simulink model "SF040A_MotVel"  (R2013b)
settings: Solver=FixedStepDiscrete  SolverMode=SingleTasking  StartTime=0.0  StopTime=1  FixedStep=6.25E-5  RelTol=1e-3
values from neighbouring files (symbols this model uses):
  ARCHGLBPRM_2MILLISEC_SEC_F32 = DataDict.Constant    [SF040A_MotVel_DataDict.m]
  ARCHGLBPRM_2PI_ULS_F32 = DataDict.Constant    [SF040A_MotVel_DataDict.m]
  ARCHGLBPRM_FLOATZEROTHD_ULS_F32 = DataDict.Constant    [SF040A_MotVel_DataDict.m]
  ARCHGLBPRM_PI_ULS_F32 = DataDict.Constant    [SF040A_MotVel_DataDict.m]
  BITMASK16BIT_CNT_U32 = DataDict.Constant    [SF040A_MotVel_DataDict.m]
  BUFSIZE_CNT_U08 = DataDict.Constant    [SF040A_MotVel_DataDict.m]
  BUFSIZECOMBD_CNT_U08 = DataDict.Constant    [SF040A_MotVel_DataDict.m]
  MOTVELMAXININVAL_CNT_U08 = DataDict.Constant    [SF040A_MotVel_DataDict.m]
  SECTOMICROSEC_ULS_F32 = DataDict.Constant    [SF040A_MotVel_DataDict.m]
  SysGlbPrmSysKineRat = DataDict.ImprtdCal    [SF040A_MotVel_DataDict.m]
libraries: simulink x7, NxtrLim x3, FixdToFloat x1
(part 1 of 2)
settings Model: Creator=BZHF94  LastModifiedBy=bzhf94
settings SolverCC: AutoInsertRateTranBlk=on  InsertRTBMode=Always
settings DataIOCC: LimitDataPoints=off  SaveFormat=Structure  ReturnWorkspaceOutputs=on
settings OptimizationCC: BlockReduction=off  InlineParams=on  ZeroExternalMemoryAtStartup=off  ZeroInternalMemoryAtStartup=off  OptimizeModelRefInitCode=on  LifeSpan=1
settings DebuggingCC: SignalInfNanChecking=error  SignalRangeChecking=warning  UnderspecifiedInitializationDetection=Simplified  SolverPrmCheckMsg=error  InheritedTsInSrcMsg=error  DiscreteInheritContinuousMsg=error  SingleTaskRateTransMsg=error  TasksWithSamePriorityMsg=error  SigSpecEnsureSampleTimeMsg=error  CheckMatrixSingularityMsg=error  ParameterUnderflowMsg=error  ParameterPrecisionLossMsg=error  ParameterTunabilityLossMsg=error  FixptConstUnderflowMsg=warning  FixptConstOverflowMsg=warning  VectorMatrixConversionMsg=error  SignalLabelMismatchMsg=error  UnconnectedInputMsg=error  UnconnectedOutputMsg=error  UnconnectedLineMsg=error  SFcnCompatibilityMsg=error  UniqueDataStoreMsg=warning  BusObjectLabelMismatch=error  RootOutportRequireBusObject=error  AssertControl=DisableAll  ModelReferenceIOMsg=error  ModelReferenceVersionMismatchMessage=warning  ModelReferenceIOMismatchMessage=error  ModelReferenceCSMismatchMessage=warning  ModelReferenceDataLoggingMessage=error  StateNameClashWarn=warning  StrictBusMsg=ErrorOnBusTreatedAsVector  NonBusSignalsTreatedAsBus=error  SFUnexpectedBacktrackingDiag=error  SFInvalidInputDataAccessInChartInitDiag=error  SFNoUnconditionalDefaultTransitionDiag=error  SFTransitionOutsideNaturalParentDiag=error  SFUnconditionalTransitionShadowingDiag=error  SFUndirectedBroadcastEventsDiag=error
settings ModelReferenceCC: ModelReferenceNumInstancesAllowed=Single
settings RTWCC: SystemTargetFile=autosar.tlc  GenCodeOnly=on  TemplateMakefile=ert_default_tmf  Description=AUTOSAR  GenerateReport=on  ProcessScript=autosar_make_rtw_hook  LaunchReport=on
settings CodeAppCC: GenerateComments=off  IgnoreCustomStorageClasses=off  CustomSymbolStrType=$N$R$M  CustomSymbolStrBlkIO=$N$M  SimulinkBlockComments=off
settings STFCustomTargetCC: ParMdlRefBuildCompliant=on  CompOptLevelCompliant=on  IncludeMdlTerminateFcn=off  CombineOutputUpdateFcns=on  SuppressErrorStatus=on  ERTFirstTimeCompliant=on  ERTCustomFileBanners=on  SupportNonFinite=off  SupportComplex=off  SupportContinuousTime=off  SupportNonInlinedSFcns=off  MATLABClassNameForMDSCustomization=Simulink.SoftwareTarget.ERTCustomization  AutosarCompliant=on  GRTInterface=off  SystemTargetFile=autosar.tlc
settings ERTTargetCC: CodeReplacementLibrary=ANSI_C  ConcurrentExecutionCompliant=off  IncludeMdlTerminateFcn=off  SuppressErrorStatus=on  SupportNonFinite=off  SupportComplex=off  ModelStepFunctionPrototypeControlCompliant=off  CPPClassGenCompliant=off  AutosarCompliant=on  InlinedParameterPlacement=NonHierarchical  ERTCustomFileTemplate=example_file_process.tlc  EnableUserReplacementTypes=on

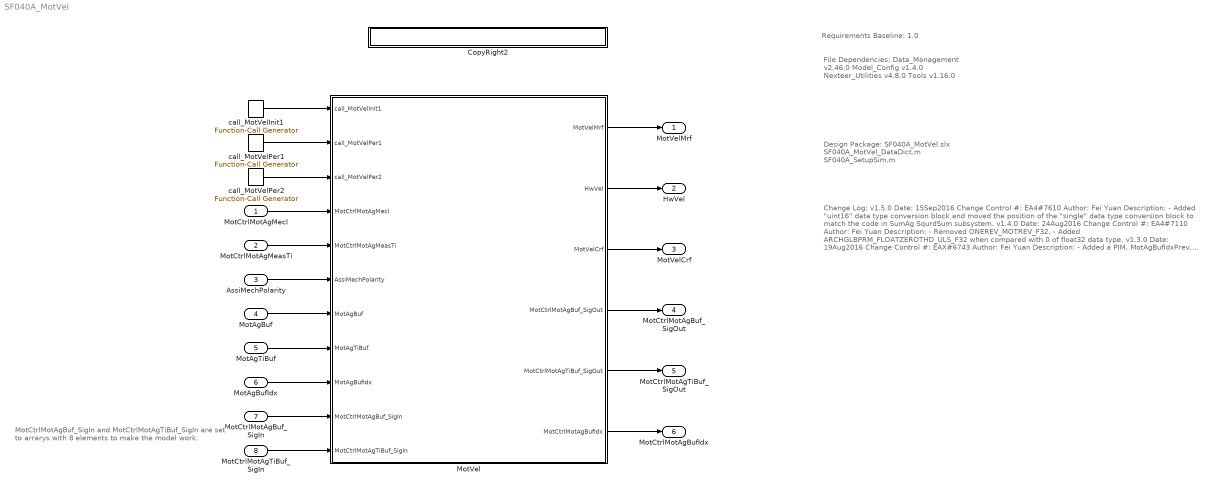
== system SF040A_MotVel ==
  note: MotCtrlMotAgBuf_SigIn and MotCtrlMotAgTiBuf_SigIn are
      | set to arrarys with 8 elements to make the model work.
  note: Change Log:
      |
      |
      | v1.5.0
      | Date: 15Sep2016
      | Change Control #: EA4#7610
      | Author: Fei Yuan
      | Description:
      | - Added "uint16" data type conversion block and moved the position of the
      |   "single" data type conversion block to match the code in SumAg SqurdSum
      |   subsystem.
      |
      | v1.4.0
      | Date: 24Aug2016
      | Change Control #: EA4#7110
      | Author: Fei Yuan
      | Description:
      | - Removed ONEREV_MOTREV_F32.
      | - Added ARCHGLBPRM_FLOATZEROTHD_ULS_F32 when compared with
      |   0 of float32 data type.
      |
      | v1.3.0
      | Date: 19Aug2016
      | Change Control #: EAX#6743
      | Author: Fei Yuan
      | Description:
      | - Added a PIM, MotAgBufIdxPrev, 3 constants, ARCHGLBPRM_PI_ULS_F32,
      |   BITCON_CNT_U32, BUFSIZE2_CNT_U08.
      | - Changed the index used for calculation MotAgRef and TiStampRef.
      | - Converted the time stamp data type from u32 to u16 before any calculation.
      | - Changed the location of conversion of MotAg from MotRev to MotRad, and
      |   MotAgTi from MicroSec to Sec.
      | - Removed constant ADJTISTAMPFAC_CNT_U08, HALFREV_MOTREV_F32.
      | - Changed constant MICROSECTOSEC_ULS_F32 to
      |    MICROSECTOSEC_ULS_F32.
      |
      |
      | v 1.2.0
      | Date: 08Jun2016
      | CR#: EA4#5936
      | Author: Fei Yuan
      | Description:
      | - Added data type conversion blocks to match the code.
      | - Changed the EngDT to u0p16 for dMotVelMotAgRef.
      | - Changed the EngDT to u0p16 and EngMax to 0.9999847412 for
      |   MotAgBufPrev.
      | - Changed the EngDT to u32 for MotAgTiBufPrev.
      | - MotCtrlMotAgBuf_SigIn and MotCtrlMotAgTiBuf_SigIn are set to
      |   arrarys with 8 elements to make the model work.
      |
      | v 1.1.0
      | Date: 13Apr2016
      | Change Control #: EA4#5282
      | Author: Fei Yuan
      | Description:
      | - Replaced MotCtrlMotAgBufPrev and MotCtrlMotAgTiBufPrev with 2 input
      |   signals, MotCtrlMotAgBuf and MotCtrlMotAgTiBuf.
      | - Moved 3 PIMs, SumTiStampBufStPrev, SumAgTiMotRevSecPrev and
      |   SqdSumTiStampPrev from the structure layer to the layer where they
      |   were used and deleted the definition in the data dictionary.
      | - Changed the PIMs names, IdxCntrPrev to MotAgBufIdx, and VelInitCntr
      |   to MotVelIninCntr.
      |
      | v 1.0.0
      | Date: 30Mar2016
      | Change Control #:  EA4#4986
      | Author: Fei Yuan
      | Description:
      |
      | - Initial release (copy over from SF040B v 1.1.0)
      | - Change the MotVelPer1.Context to 'Non-Rte' and MotVelPer1.TimeStep
      |   to 'MotorControl'.
      | - Change the EngInit of MotAgBuf, MotAgTiBuf
  note: File Dependencies:
      |
      | Data_Management v2.46.0
      | Model_Config v1.4.0
      | Nexteer_Utilities v4.8.0
      | Tools v1.16.0
  note: Requirements Baseline: 1.0
  note: Design Package:
      | SF040A_MotVel.slx
      | SF040A_MotVel_DataDict.m
      | SF040A_SetupSim.m
  MotCtrlMotAgMecl : Inport
  MotCtrlMotAgMeasTi : Inport  Port=2
  AssiMechPolarity : Inport  Port=3
  MotAgBuf : Inport  Port=4
  MotAgTiBuf : Inport  Port=5
  MotAgBufIdx : Inport  Port=6
  MotCtrlMotAgBuf_SigIn : Inport  Port=7  PortDimensions=8
  MotCtrlMotAgTiBuf_SigIn : Inport  Port=8  PortDimensions=8
  CopyRight2 : Subsystem  Description=|  mask(Copyright Information){none=on}
      | Copyright info block.                                               
      |                                                                     
      | Place copyright information at the top of every subsystem in design.
      mask prompts: none "No parameters"
      mask help: Place copyright information at the top of every subsystem in design.
      mask Display:
      | NxtrConf = 'Nexteer Confidential';
      | 
      | sys = bdroot; %handle for the current model ("system")
      | first = get_param(sys,'Created');
      | first = first(end-3:end);  %year is last four digits
      | 
      | last = get_param(sys,'LastModifiedDate');
      | if isempty(last)
      |     last = datestr(now,'yyyy');
      | else
      |     last = last(end-3:end);
      | end
      | 
      | if strcmp(first,last)
      |     fprintf('%s -- Copyright %s Nexteer',NxtrConf,first)
      | else
      |     fprintf('%s -- %s%s- %s Nexteer',NxtrConf,char(169),first,last)
      | end
  MotVel : Subsystem
  call_MotVelInit1 : simulink/Ports & Subsystems/Function-Call Generator  sample_time=0.002  numberOfIterations=1
  call_MotVelPer1 : simulink/Ports & Subsystems/Function-Call Generator  sample_time=0.0000625  numberOfIterations=1
  call_MotVelPer2 : simulink/Ports & Subsystems/Function-Call Generator  sample_time=.002  numberOfIterations=1
  MotVelMrf : Outport
  HwVel : Outport  Port=2
  MotVelCrf : Outport  Port=3
  MotCtrlMotAgBuf_SigOut : Outport  Port=4
  MotCtrlMotAgTiBuf_SigOut : Outport  Port=5
  MotCtrlMotAgBufIdx : Outport  Port=6
  wires:
  MotVel/1(MotVelMrf) -> MotVelMrf/1
  MotVel/2(HwVel) -> HwVel/1
  MotVel/3(MotVelCrf) -> MotVelCrf/1
  MotVel/4(MotCtrlMotAgBuf_SigOut) -> MotCtrlMotAgBuf_SigOut/1
  MotVel/5(MotCtrlMotAgTiBuf_SigOut) -> MotCtrlMotAgTiBuf_SigOut/1
  call_MotVelInit1/1 -> MotVel/1(call_MotVelInit1)
  call_MotVelPer1/1 -> MotVel/2(call_MotVelPer1)
  call_MotVelPer2/1 -> MotVel/3(call_MotVelPer2)
  MotCtrlMotAgMecl/1 -> MotVel/4(MotCtrlMotAgMecl)
  MotCtrlMotAgMeasTi/1 -> MotVel/5(MotCtrlMotAgMeasTi)
  MotAgBufIdx/1 -> MotVel/9(MotAgBufIdx)
  AssiMechPolarity/1 -> MotVel/6(AssiMechPolarity)
  MotVel/6(MotCtrlMotAgBufIdx) -> MotCtrlMotAgBufIdx/1
  MotCtrlMotAgBuf_SigIn/1 -> MotVel/10(MotCtrlMotAgBuf_SigIn)
  MotCtrlMotAgTiBuf_SigIn/1 -> MotVel/11(MotCtrlMotAgTiBuf_SigIn)
  MotAgBuf/1 -> MotVel/7(MotAgBuf)
  MotAgTiBuf/1 -> MotVel/8(MotAgTiBuf)

== system SF040A_MotVel/CopyRight2 ==

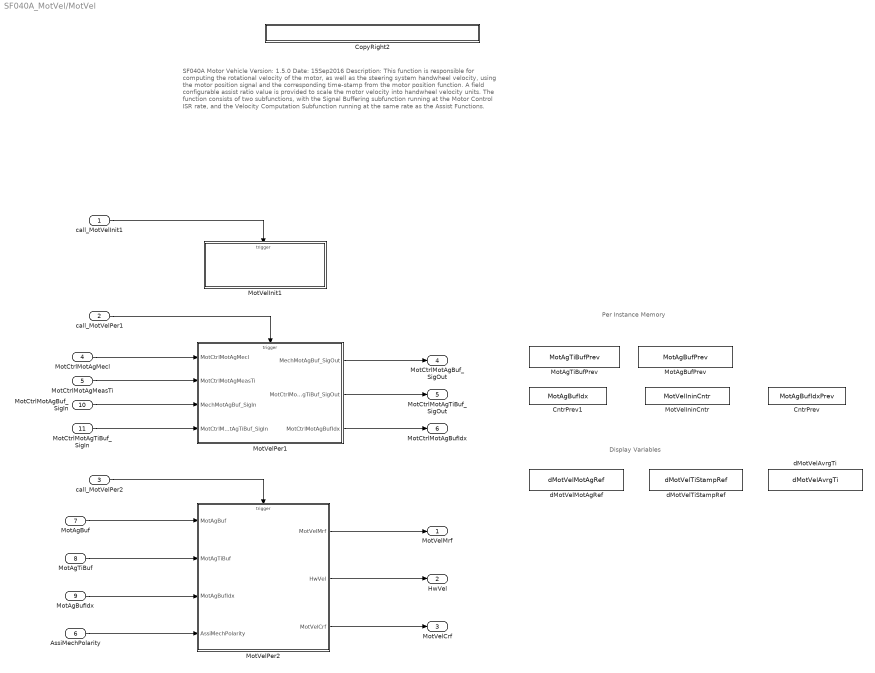
== system SF040A_MotVel/MotVel ==
  note: Display Variables
  note: Per Instance Memory
  note: SF040A Motor Vehicle
      | Version: 1.5.0							Date: 15Sep2016
      |
      | Description:
      | This function is responsible for computing the rotational velocity of the motor, as well as the steering system handwheel velocity,
      | using the motor position signal and the corresponding time-stamp from the motor position function.  A field configurable assist
      | ratio value is provided to scale the motor velocity into handwheel velocity units.  The function consists of two subfunctions, with
      | the Signal Buffering subfunction running at the Motor Control ISR rate, and the Velocity Computation Subfunction running at the
      | same rate as the Assist Functions.
  call_MotVelInit1 : Inport
  call_MotVelPer1 : Inport  RequirementInfo="{'linktype_rmi_doors' '0000bab8 (/E-STEER Core/SubSystem Specifications/Application Functions/SF040A Motor Velocity)' '#SF040A_100' 'true' 'REQ:  SF040A_100' '' } %GIDa_c56390ee_26f7_4798_9213_76a7503bffac"  Port=2
  call_MotVelPer2 : Inport  RequirementInfo="{'linktype_rmi_doors' '0000bab8 (/E-STEER Core/SubSystem Specifications/Application Functions/SF040A Motor Velocity)' '#SF040A_101' 'true' 'REQ:  SF040A_101' '' } %GIDa_45187939_3049_4216_a5ff_224b0e3b0d5f"  Port=3
  MotCtrlMotAgMecl : Inport  RequirementInfo="{'linktype_rmi_doors' '0000bab8 (/E-STEER Core/SubSystem Specifications/Application Functions/SF040A Motor Velocity)' '#SF040A_9' 'true' 'REQ:  SF040A_9' '' } %GIDa_da6e85f8_c467_48fd_86b9_994a95a2d77e"  Port=4
  MotCtrlMotAgMeasTi : Inport  RequirementInfo="{'linktype_rmi_doors' '0000bab8 (/E-STEER Core/SubSystem Specifications/Application Functions/SF040A Motor Velocity)' '#SF040A_32' 'true' 'REQ:  SF040A_32' '' } %GIDa_271797b2_38a6_4cdb_aa6b_2c4163c3e0fb"  Port=5
  AssiMechPolarity : Inport  RequirementInfo="{'linktype_rmi_doors' '0000bab8 (/E-STEER Core/SubSystem Specifications/Application Functions/SF040A Motor Velocity)' '#SF040A_67' 'true' 'REQ:  SF040A_67' '' } %GIDa_5dcd69b4_bba5_4e51_813a_ddc0e3c93255"  Port=6
  MotAgBuf : Inport  RequirementInfo="{'linktype_rmi_doors' '0000bab8 (/E-STEER Core/SubSystem Specifications/Application Functions/SF040A Motor Velocity)' '#SF040A_37' 'true' 'REQ:  SF040A_37' '' } %GIDa_7b59af74_1f9f_4213_9473_c6c052ccc2e7"  Port=7
  MotAgTiBuf : Inport  RequirementInfo="{'linktype_rmi_doors' '0000bab8 (/E-STEER Core/SubSystem Specifications/Application Functions/SF040A Motor Velocity)' '#SF040A_38' 'true' 'REQ:  SF040A_38' '' } %GIDa_7f2c140d_1132_4c80_bf72_e1f2d4b4c4b3"  Port=8
  MotAgBufIdx : Inport  RequirementInfo="{'linktype_rmi_doors' '0000bab8 (/E-STEER Core/SubSystem Specifications/Application Functions/SF040A Motor Velocity)' '#SF040A_68' 'true' 'REQ:  SF040A_68' '' } %GIDa_6a748ccc_0dcc_4377_8e15_da7874ab802e"  Port=9
  MotCtrlMotAgBuf_SigIn : Inport  Port=10
  MotCtrlMotAgTiBuf_SigIn : Inport  Port=11
  CntrPrev : DataStoreMemory  DataStoreName=MotAgBufIdxPrev  InitialValue=[]  StateMustResolveToSignalObject=on
  CntrPrev1 : DataStoreMemory  DataStoreName=MotAgBufIdx  InitialValue=[]  StateMustResolveToSignalObject=on
  CopyRight2 : Subsystem  Description=|  mask(Copyright Information){none=on}
      | Copyright info block.                                               
      |                                                                     
      | Place copyright information at the top of every subsystem in design.
      mask prompts: none "No parameters"
      mask help: Place copyright information at the top of every subsystem in design.
      mask Display:
      | NxtrConf = 'Nexteer Confidential';
      | 
      | sys = bdroot; %handle for the current model ("system")
      | first = get_param(sys,'Created');
      | first = first(end-3:end);  %year is last four digits
      | 
      | last = get_param(sys,'LastModifiedDate');
      | if isempty(last)
      |     last = datestr(now,'yyyy');
      | else
      |     last = last(end-3:end);
      | end
      | 
      | if strcmp(first,last)
      |     fprintf('%s -- Copyright %s Nexteer',NxtrConf,first)
      | else
      |     fprintf('%s -- %s%s- %s Nexteer',NxtrConf,char(169),first,last)
      | end
  MotAgBufPrev : DataStoreMemory  DataStoreName=MotAgBufPrev  InitialValue=[]  StateMustResolveToSignalObject=on
  MotAgTiBufPrev : DataStoreMemory  DataStoreName=MotAgTiBufPrev  InitialValue=[]  StateMustResolveToSignalObject=on
  MotVelIninCntr : DataStoreMemory  DataStoreName=MotVelIninCntr  StateMustResolveToSignalObject=on
  MotVelInit1 : Subsystem  Tag=Oversampling and Buffering
  MotVelPer1 : Subsystem  Tag=Oversampling and Buffering  RequirementInfo={} %GIDa_d50e150f_09b9_4d8d_ad89_b52fa6920a08
  MotVelPer2 : Subsystem  Tag=Motor Velocity Main Function  RequirementInfo={} %GIDa_2064eca6_58da_4904_baf1_7d9f427526b9
  dMotVelAvrgTi : DataStoreMemory  DataStoreName=dMotVelAvrgTi  StateMustResolveToSignalObject=on
  dMotVelMotAgRef : DataStoreMemory  DataStoreName=dMotVelMotAgRef  StateMustResolveToSignalObject=on
  dMotVelTiStampRef : DataStoreMemory  DataStoreName=dMotVelTiStampRef  StateMustResolveToSignalObject=on
  MotVelMrf : Outport  RequirementInfo="{'linktype_rmi_doors' '0000bab8 (/E-STEER Core/SubSystem Specifications/Application Functions/SF040A Motor Velocity)' '#SF040A_43' 'true' 'REQ:  SF040A_43' '' } %GIDa_fb85c017_91e0_421c_ab95_15c37d20c5e7"
  HwVel : Outport  RequirementInfo="{'linktype_rmi_doors' '0000bab8 (/E-STEER Core/SubSystem Specifications/Application Functions/SF040A Motor Velocity)' '#SF040A_45' 'true' 'REQ:  SF040A_45' '' } %GIDa_6b0f4a8b_2a28_46b6_aefd_175b69bc11de"  Port=2
  MotVelCrf : Outport  RequirementInfo="{'linktype_rmi_doors' '0000bab8 (/E-STEER Core/SubSystem Specifications/Application Functions/SF040A Motor Velocity)' '#SF040A_44' 'true' 'REQ:  SF040A_44' '' } %GIDa_094eba48_af1d_4fc7_b429_5fbb699d5d26"  Port=3
  MotCtrlMotAgBuf_SigOut : Outport  RequirementInfo="{'linktype_rmi_doors' '0000bab8 (/E-STEER Core/SubSystem Specifications/Application Functions/SF040A Motor Velocity)' '#SF040A_11' 'true' 'REQ:  SF040A_11' '' } %GIDa_1d8b269e_d694_4cbb_9508_c106a0fbc47a"  Port=4
  MotCtrlMotAgTiBuf_SigOut : Outport  RequirementInfo="{'linktype_rmi_doors' '0000bab8 (/E-STEER Core/SubSystem Specifications/Application Functions/SF040A Motor Velocity)' '#SF040A_39' 'true' 'REQ:  SF040A_39' '' } %GIDa_a0bee6bf_8359_42f0_986c_befce60871f1"  Port=5
  MotCtrlMotAgBufIdx : Outport  RequirementInfo="{'linktype_rmi_doors' '0000bab8 (/E-STEER Core/SubSystem Specifications/Application Functions/SF040A Motor Velocity)' '#SF040A_40' 'true' 'REQ:  SF040A_40' '' } %GIDa_e6a0b20c_cb09_47a3_9c37_aa599aec0d6b"  Port=6
  wires:
  MotCtrlMotAgMecl/1 -> MotVelPer1/1(MotCtrlMotAgMecl)
  MotVelPer2/1(MotVelMrf) -> MotVelMrf/1
  MotVelPer2/2(HwVel) -> HwVel/1
  MotCtrlMotAgMeasTi/1 -> MotVelPer1/2(MotCtrlMotAgMeasTi)
  MotVelPer2/3(MotVelCrf) -> MotVelCrf/1
  MotVelPer1/1(MechMotAgBuf_SigOut) -> MotCtrlMotAgBuf_SigOut/1
  MotVelPer1/2(MotCtrlMotAgTiBuf_SigOut) -> MotCtrlMotAgTiBuf_SigOut/1
  call_MotVelPer1/1 -> MotVelPer1/Trigger
  call_MotVelPer2/1 -> MotVelPer2/Trigger
  AssiMechPolarity/1 -> MotVelPer2/4(AssiMechPolarity)
  MotAgTiBuf/1 -> MotVelPer2/2(MotAgTiBuf)
  MotAgBuf/1 -> MotVelPer2/1(MotAgBuf)
  MotAgBufIdx/1 -> MotVelPer2/3(MotAgBufIdx)
  call_MotVelInit1/1 -> MotVelInit1/Trigger
  MotVelPer1/3(MotCtrlMotAgBufIdx) -> MotCtrlMotAgBufIdx/1
  MotCtrlMotAgBuf_SigIn/1 -> MotVelPer1/3(MechMotAgBuf_SigIn)
  MotCtrlMotAgTiBuf_SigIn/1 -> MotVelPer1/4(MotCtrlMotAgTiBuf_SigIn)

== system SF040A_MotVel/MotVel/CopyRight2 ==

== system SF040A_MotVel/MotVel/MotVelInit1 ==
  note: /*Do Nothing*/
  function : TriggerPort  TriggerType=function-call
  CopyRight2 : Subsystem  Description=|  mask(Copyright Information){none=on}
      | Copyright info block.                                               
      |                                                                     
      | Place copyright information at the top of every subsystem in design.
      mask prompts: none "No parameters"
      mask help: Place copyright information at the top of every subsystem in design.
      mask Display:
      | NxtrConf = 'Nexteer Confidential';
      | 
      | sys = bdroot; %handle for the current model ("system")
      | first = get_param(sys,'Created');
      | first = first(end-3:end);  %year is last four digits
      | 
      | last = get_param(sys,'LastModifiedDate');
      | if isempty(last)
      |     last = datestr(now,'yyyy');
      | else
      |     last = last(end-3:end);
      | end
      | 
      | if strcmp(first,last)
      |     fprintf('%s -- Copyright %s Nexteer',NxtrConf,first)
      | else
      |     fprintf('%s -- %s%s- %s Nexteer',NxtrConf,char(169),first,last)
      | end

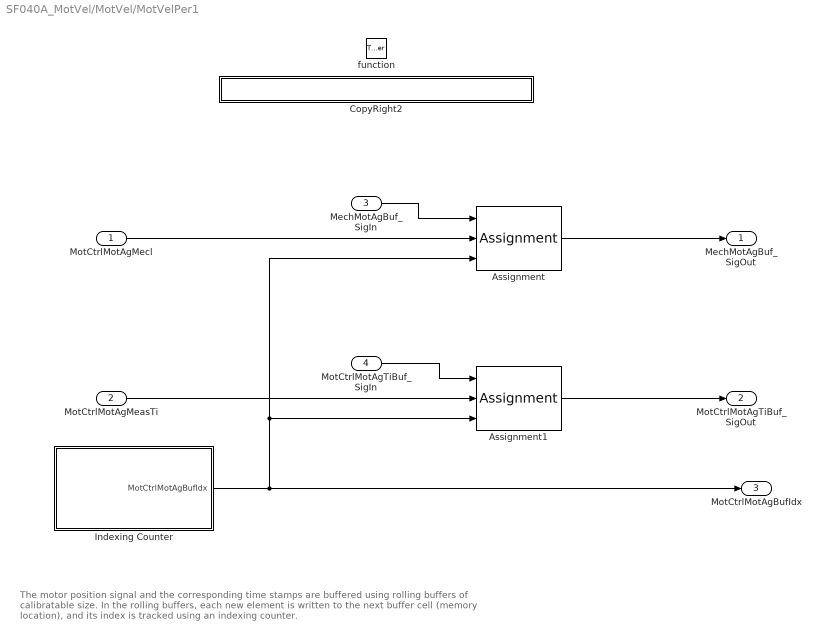
== system SF040A_MotVel/MotVel/MotVelPer1 ==
  note: The motor position signal and the corresponding time stamps are buffered using rolling buffers of calibratable size.
      | In the rolling buffers, each new element is written to the next buffer cell (memory location), and its index is tracked
      | using an indexing counter.
  MotCtrlMotAgMecl : Inport
  MotCtrlMotAgMeasTi : Inport  Port=2
  MechMotAgBuf_SigIn : Inport  Port=3
  MotCtrlMotAgTiBuf_SigIn : Inport  Port=4
  function : TriggerPort  TriggerType=function-call
  Assignment : Assignment  RequirementInfo="{'linktype_rmi_doors' '0000bab8 (/E-STEER Core/SubSystem Specifications/Application Functions/SF040A Motor Velocity)' '#SF040A_75' 'true' 'REQ:  SF040A_75' '' } %GIDa_ba215c0f_c2e7_45a4_8c50_a26cb4d5c437"  IndexMode=Zero-based  IndexOptions=Index vector (port)  Indices=1  OutputSizes=1
  Assignment1 : Assignment  RequirementInfo="{'linktype_rmi_doors' '0000bab8 (/E-STEER Core/SubSystem Specifications/Application Functions/SF040A Motor Velocity)' '#SF040A_77' 'true' 'REQ:  SF040A_77' '' } %GIDa_f38257c3_ca74_4bda_804f_05d76b61db45"  IndexMode=Zero-based  IndexOptions=Index vector (port)  Indices=1  OutputSizes=1
  CopyRight2 : Subsystem  Description=|  mask(Copyright Information){none=on}
      | Copyright info block.                                               
      |                                                                     
      | Place copyright information at the top of every subsystem in design.
      mask prompts: none "No parameters"
      mask help: Place copyright information at the top of every subsystem in design.
      mask Display:
      | NxtrConf = 'Nexteer Confidential';
      | 
      | sys = bdroot; %handle for the current model ("system")
      | first = get_param(sys,'Created');
      | first = first(end-3:end);  %year is last four digits
      | 
      | last = get_param(sys,'LastModifiedDate');
      | if isempty(last)
      |     last = datestr(now,'yyyy');
      | else
      |     last = last(end-3:end);
      | end
      | 
      | if strcmp(first,last)
      |     fprintf('%s -- Copyright %s Nexteer',NxtrConf,first)
      | else
      |     fprintf('%s -- %s%s- %s Nexteer',NxtrConf,char(169),first,last)
      | end
  Indexing Counter : Subsystem  RequirementInfo="{'linktype_rmi_doors' '0000bab8 (/E-STEER Core/SubSystem Specifications/Application Functions/SF040A Motor Velocity)' '#SF040A_76' 'true' 'REQ:  SF040A_76' '' } %GIDa_4ec6e91e_0e82_4c5e_a61d_983bd7ddc339"
  MechMotAgBuf_SigOut : Outport
  MotCtrlMotAgTiBuf_SigOut : Outport  Port=2
  MotCtrlMotAgBufIdx : Outport  Port=3
  wires:
  Indexing Counter/1(MotCtrlMotAgBufIdx) -> MotCtrlMotAgBufIdx/1, Assignment1/3, Assignment/3
  Assignment/1 -> MechMotAgBuf_SigOut/1
  MechMotAgBuf_SigIn/1 -> Assignment/1
  Assignment1/1 -> MotCtrlMotAgTiBuf_SigOut/1
  MotCtrlMotAgTiBuf_SigIn/1 -> Assignment1/1
  MotCtrlMotAgMecl/1 -> Assignment/2
  MotCtrlMotAgMeasTi/1 -> Assignment1/2

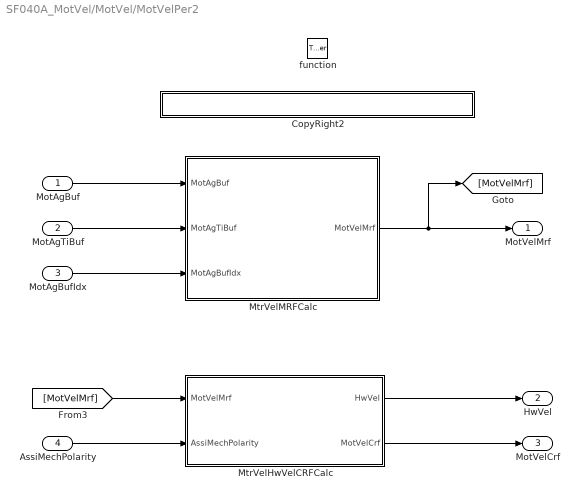
== system SF040A_MotVel/MotVel/MotVelPer2 ==
  MotAgBuf : Inport
  MotAgTiBuf : Inport  Port=2
  MotAgBufIdx : Inport  Port=3
  AssiMechPolarity : Inport  Port=4
  function : TriggerPort  TriggerType=function-call
  CopyRight2 : Subsystem  Description=|  mask(Copyright Information){none=on}
      | Copyright info block.                                               
      |                                                                     
      | Place copyright information at the top of every subsystem in design.
      mask prompts: none "No parameters"
      mask help: Place copyright information at the top of every subsystem in design.
      mask Display:
      | NxtrConf = 'Nexteer Confidential';
      | 
      | sys = bdroot; %handle for the current model ("system")
      | first = get_param(sys,'Created');
      | first = first(end-3:end);  %year is last four digits
      | 
      | last = get_param(sys,'LastModifiedDate');
      | if isempty(last)
      |     last = datestr(now,'yyyy');
      | else
      |     last = last(end-3:end);
      | end
      | 
      | if strcmp(first,last)
      |     fprintf('%s -- Copyright %s Nexteer',NxtrConf,first)
      | else
      |     fprintf('%s -- %s%s- %s Nexteer',NxtrConf,char(169),first,last)
      | end
  MtrVelHwVelCRFCalc : Subsystem  Tag=Motor and Handwheel Velocity Calculation in CRF  RequirementInfo={} %GIDa_f0326ab6_3913_4c0f_a6ed_180ca0f254da
      settings: AttributesFormatString=%<Tag>
  MtrVelMRFCalc : Subsystem  Tag=Motor Velocity Calculation  RequirementInfo={} %GIDa_d0edbfbb_9837_4dd6_ba84_42533fbd77e9
  MotVelMrf : Outport  RequirementInfo={} %GIDa_9ad7ed95_999a_48b5_95cd_2dea3e6a19bc
  HwVel : Outport  RequirementInfo={} %GIDa_4e8b83db_f51a_4af5_ab52_7c1be925920f  Port=2
  MotVelCrf : Outport  RequirementInfo={} %GIDa_28b0c72c_8b37_40d4_83ce_e69512ee35c8  Port=3
  wires:
  MtrVelMRFCalc/1(MotVelMrf) -> [MotVelMrf], MotVelMrf/1
  MtrVelHwVelCRFCalc/1(HwVel) -> HwVel/1
  MtrVelHwVelCRFCalc/2(MotVelCrf) -> MotVelCrf/1
  [MotVelMrf] -> MtrVelHwVelCRFCalc/1(MotVelMrf)
  AssiMechPolarity/1 -> MtrVelHwVelCRFCalc/2(AssiMechPolarity)
  MotAgTiBuf/1 -> MtrVelMRFCalc/2(MotAgTiBuf)
  MotAgBuf/1 -> MtrVelMRFCalc/1("MotAgBuf ")
  MotAgBufIdx/1 -> MtrVelMRFCalc/3(MotAgBufIdx)

== system SF040A_MotVel/MotVel/MotVelInit1/CopyRight2 ==

== system SF040A_MotVel/MotVel/MotVelPer1/CopyRight2 ==

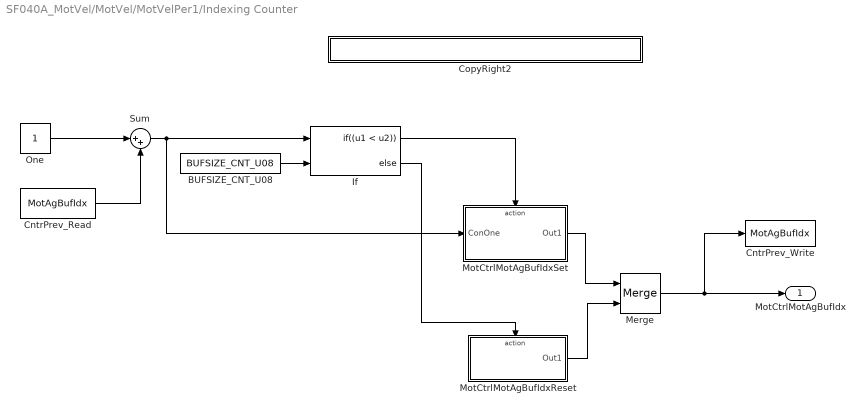
== system SF040A_MotVel/MotVel/MotVelPer1/Indexing Counter ==
  BUFSIZE_CNT_U08 : Constant  Value=BUFSIZE_CNT_U08  OutDataTypeStr=Inherit: Inherit via back propagation
  CntrPrev_Read : DataStoreRead  DataStoreName=MotAgBufIdx
  CntrPrev_Write : DataStoreWrite  DataStoreName=MotAgBufIdx
  CopyRight2 : Subsystem  Description=|  mask(Copyright Information){none=on}
      | Copyright info block.                                               
      |                                                                     
      | Place copyright information at the top of every subsystem in design.
      mask prompts: none "No parameters"
      mask help: Place copyright information at the top of every subsystem in design.
      mask Display:
      | NxtrConf = 'Nexteer Confidential';
      | 
      | sys = bdroot; %handle for the current model ("system")
      | first = get_param(sys,'Created');
      | first = first(end-3:end);  %year is last four digits
      | 
      | last = get_param(sys,'LastModifiedDate');
      | if isempty(last)
      |     last = datestr(now,'yyyy');
      | else
      |     last = last(end-3:end);
      | end
      | 
      | if strcmp(first,last)
      |     fprintf('%s -- Copyright %s Nexteer',NxtrConf,first)
      | else
      |     fprintf('%s -- %s%s- %s Nexteer',NxtrConf,char(169),first,last)
      | end
  If : If  NumInputs=2  IfExpression=(u1 < u2)
  Merge : Merge
  MotCtrlMotAgBufIdxReset : Subsystem  TreatAsAtomicUnit=on
  MotCtrlMotAgBufIdxSet : Subsystem  TreatAsAtomicUnit=on
  One : Constant  OutDataTypeStr=Inherit: Inherit via back propagation
  Sum : Sum  Inputs=|++
  MotCtrlMotAgBufIdx : Outport
  wires:
  BUFSIZE_CNT_U08/1 -> If/2
  One/1 -> Sum/1
  CntrPrev_Read/1 -> Sum/2
  Sum/1 -> If/1, MotCtrlMotAgBufIdxSet/1(ConOne)
  MotCtrlMotAgBufIdxSet/1(Out1) -> Merge/1
  Merge/1 -> CntrPrev_Write/1, MotCtrlMotAgBufIdx/1
  MotCtrlMotAgBufIdxReset/1(Out1) -> Merge/2
  If/1 -> MotCtrlMotAgBufIdxSet/Action
  If/2 -> MotCtrlMotAgBufIdxReset/Action

== system SF040A_MotVel/MotVel/MotVelPer2/CopyRight2 ==

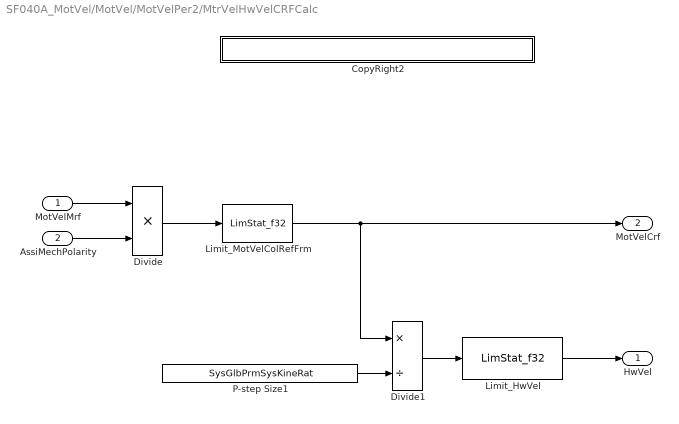
== system SF040A_MotVel/MotVel/MotVelPer2/MtrVelHwVelCRFCalc ==
  MotVelMrf : Inport
  AssiMechPolarity : Inport  Port=2
  CopyRight2 : Subsystem  Description=|  mask(Copyright Information){none=on}
      | Copyright info block.                                               
      |                                                                     
      | Place copyright information at the top of every subsystem in design.
      mask prompts: none "No parameters"
      mask help: Place copyright information at the top of every subsystem in design.
      mask Display:
      | NxtrConf = 'Nexteer Confidential';
      | 
      | sys = bdroot; %handle for the current model ("system")
      | first = get_param(sys,'Created');
      | first = first(end-3:end);  %year is last four digits
      | 
      | last = get_param(sys,'LastModifiedDate');
      | if isempty(last)
      |     last = datestr(now,'yyyy');
      | else
      |     last = last(end-3:end);
      | end
      | 
      | if strcmp(first,last)
      |     fprintf('%s -- Copyright %s Nexteer',NxtrConf,first)
      | else
      |     fprintf('%s -- %s%s- %s Nexteer',NxtrConf,char(169),first,last)
      | end
  Divide : Product  RequirementInfo="{'linktype_rmi_doors' '0000bab8 (/E-STEER Core/SubSystem Specifications/Application Functions/SF040A Motor Velocity)' '#SF040A_88' 'true' 'REQ:  SF040A_88' '' } %GIDa_d0253a6d_4a51_4c17_bca3_2bbc9e34fe30"
  Divide1 : Product  RequirementInfo="{'linktype_rmi_doors' '0000bab8 (/E-STEER Core/SubSystem Specifications/Application Functions/SF040A Motor Velocity)' '#SF040A_90' 'true' 'REQ:  SF040A_90' '' } %GIDa_14855bd5_ba8c_4be9_94d5_ae8fd5da5cfe"  Inputs=*/
  Limit_HwVel : NxtrLim/LimStat_f32  RequirementInfo="{'linktype_rmi_doors' '0000bab8 (/E-STEER Core/SubSystem Specifications/Application Functions/SF040A Motor Velocity)' '#SF040A_92' 'true' 'REQ:  SF040A_92' '' ; 'linktype_rmi_doors' '0000bab8 (/E-STEER Core/SubSystem Specifications/Application Functions/SF040A Motor Velocity)' '#SF040A_94' 'true' 'REQ:  SF040A_94' '' } %GIDa_fbda6fa3_a00d_4c12_b82e_fa73d83fe949"  LoLim=HWVELMIN_HWRADPERSEC_F32  HiLim=HWVELMAX_HWRADPERSEC_F32
      settings: AttributesFormatString=|
      | Low Limit: %<LoLim>
      | High Limit:%<HiLim>
  Limit_MotVelColRefFrm : NxtrLim/LimStat_f32  RequirementInfo="{'linktype_rmi_doors' '0000bab8 (/E-STEER Core/SubSystem Specifications/Application Functions/SF040A Motor Velocity)' '#SF040A_89' 'true' 'REQ:  SF040A_89' '' ; 'linktype_rmi_doors' '0000bab8 (/E-STEER Core/SubSystem Specifications/Application Functions/SF040A Motor Velocity)' '#SF040A_93' 'true' 'REQ:  SF040A_93' '' } %GIDa_57e8be59_5c0d_40e4_830f_d469115c4d15"  LoLim=MOTVELMIN_MOTRADPERSEC_F32  HiLim=MOTVELMAX_MOTRADPERSEC_F32
      settings: AttributesFormatString=|
      | Low Limit: %<LoLim>
      | High Limit:%<HiLim>
  P-step Size1 : Constant  RequirementInfo={} %GIDa_2f3ad8d2_2bd3_4754_bfb4_444af07a73fa  Value=SysGlbPrmSysKineRat
  HwVel : Outport
  MotVelCrf : Outport  Port=2
  wires:
  AssiMechPolarity/1 -> Divide/2
  MotVelMrf/1 -> Divide/1
  Divide/1 -> Limit_MotVelColRefFrm/1
  Divide1/1 -> Limit_HwVel/1
  P-step Size1/1 -> Divide1/2
  Limit_MotVelColRefFrm/1 -> MotVelCrf/1, Divide1/1
  Limit_HwVel/1 -> HwVel/1

== system SF040A_MotVel/MotVel/MotVelPer2/MtrVelMRFCalc ==
  "MotAgBuf " : Inport
  MotAgTiBuf : Inport  Port=2
  MotAgBufIdx : Inport  Port=3
  CopyRight2 : Subsystem  Description=|  mask(Copyright Information){none=on}
      | Copyright info block.                                               
      |                                                                     
      | Place copyright information at the top of every subsystem in design.
      mask prompts: none "No parameters"
      mask help: Place copyright information at the top of every subsystem in design.
      mask Display:
      | NxtrConf = 'Nexteer Confidential';
      | 
      | sys = bdroot; %handle for the current model ("system")
      | first = get_param(sys,'Created');
      | first = first(end-3:end);  %year is last four digits
      | 
      | last = get_param(sys,'LastModifiedDate');
      | if isempty(last)
      |     last = datestr(now,'yyyy');
      | else
      |     last = last(end-3:end);
      | end
      | 
      | if strcmp(first,last)
      |     fprintf('%s -- Copyright %s Nexteer',NxtrConf,first)
      | else
      |     fprintf('%s -- %s%s- %s Nexteer',NxtrConf,char(169),first,last)
      | end
  MtrVelMRFCalc : Subsystem
  MotVelMrf : Outport
  wires:
  MtrVelMRFCalc/1(MotVelMrf) -> MotVelMrf/1
  MotAgBufIdx/1 -> MtrVelMRFCalc/3(MotAgBufIdx)
  MotAgTiBuf/1 -> MtrVelMRFCalc/2(MotAgTiBuf)
  "MotAgBuf "/1 -> MtrVelMRFCalc/1("MotAgBuf ")

== system SF040A_MotVel/MotVel/MotVelPer1/Indexing Counter/CopyRight2 ==

== system SF040A_MotVel/MotVel/MotVelPer1/Indexing Counter/MotCtrlMotAgBufIdxReset ==
  Action Port : ActionPort  ActionType=else
  Copyright1 : Subsystem  Description=|  RequirementInfo={} %GIDa_d1bef53a_ef53_4856_b0f6_82ae1dc9e7f9  mask(Copyright Information){none=on}
      | Copyright info block.                                               
      |                                                                     
      | Place copyright information at the top of every subsystem in design.
      mask prompts: none "No parameters"
      mask help: Place copyright information at the top of every subsystem in design.
      mask Display:
      | NxtrConf = 'Nexteer Confidential';
      | 
      | sys = bdroot; %handle for the current model ("system")
      | first = get_param(sys,'Created');
      | if(isempty(first))
      |     first = datestr(now,'yyyy');
      | else
      |     first = first(end-3:end);  %year is last four digits
      | end
      | 
      | last = get_param(sys,'LastModifiedDate');
      | if isempty(last)
      |     last = datestr(now,'yyyy');
      | else
      |     last = last(end-3:end);
      | end
      | 
      | if strcmp(first,last)
      |     fprintf('%s\nCopyright  %s Nexteer',NxtrConf,first);
      | else
      |     fprintf('%s\n%s%s-%s Nexteer',NxtrConf,char(169),first,last);
      | end
  Zero : Constant  Value=0  OutDataTypeStr=Inherit: Inherit via back propagation
  Out1 : Outport
  wires:
  Zero/1 -> Out1/1

== system SF040A_MotVel/MotVel/MotVelPer1/Indexing Counter/MotCtrlMotAgBufIdxSet ==
  ConOne : Inport
  Action Port : ActionPort  ActionType=then
  Copyright1 : Subsystem  Description=|  RequirementInfo={} %GIDa_ff0b4898_c16a_43d9_8b3d_1b56a2308ffd  mask(Copyright Information){none=on}
      | Copyright info block.                                               
      |                                                                     
      | Place copyright information at the top of every subsystem in design.
      mask prompts: none "No parameters"
      mask help: Place copyright information at the top of every subsystem in design.
      mask Display:
      | NxtrConf = 'Nexteer Confidential';
      | 
      | sys = bdroot; %handle for the current model ("system")
      | first = get_param(sys,'Created');
      | if(isempty(first))
      |     first = datestr(now,'yyyy');
      | else
      |     first = first(end-3:end);  %year is last four digits
      | end
      | 
      | last = get_param(sys,'LastModifiedDate');
      | if isempty(last)
      |     last = datestr(now,'yyyy');
      | else
      |     last = last(end-3:end);
      | end
      | 
      | if strcmp(first,last)
      |     fprintf('%s\nCopyright  %s Nexteer',NxtrConf,first);
      | else
      |     fprintf('%s\n%s%s-%s Nexteer',NxtrConf,char(169),first,last);
      | end
  Out1 : Outport
  wires:
  ConOne/1 -> Out1/1

== system SF040A_MotVel/MotVel/MotVelPer2/MtrVelHwVelCRFCalc/CopyRight2 ==

== system SF040A_MotVel/MotVel/MotVelPer2/MtrVelMRFCalc/CopyRight2 ==

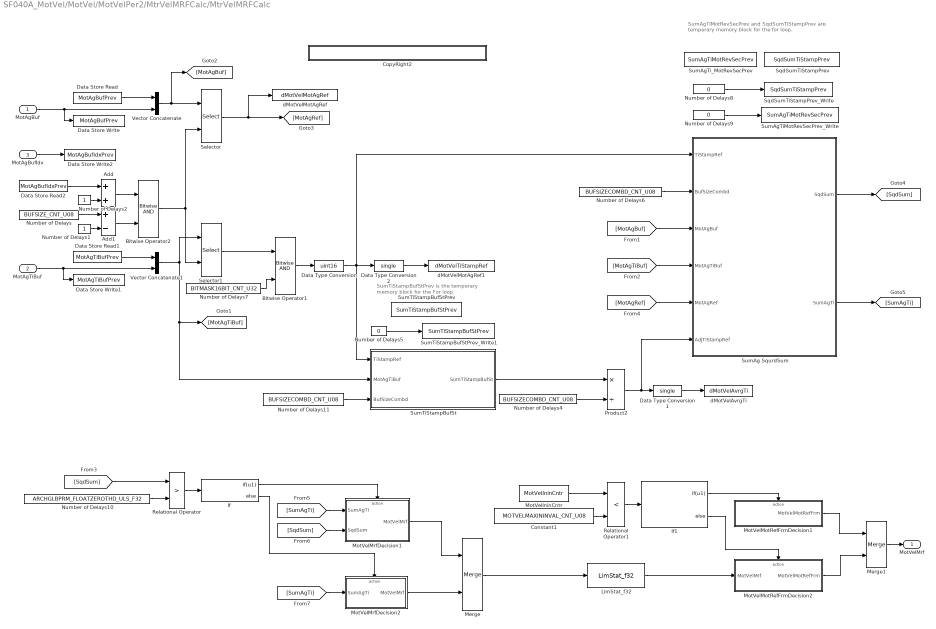
== system SF040A_MotVel/MotVel/MotVelPer2/MtrVelMRFCalc/MtrVelMRFCalc ==
  note: SumTiStampBufStPrev is the temperary
      | memory block for the For loop.
  note: SumAgTiMotRevSecPrev and SqdSumTiStampPrev are
      | temperary memory block for the for loop.
  "MotAgBuf " : Inport
  MotAgTiBuf : Inport  Port=2
  MotAgBufIdx : Inport  Port=3
  Add : Sum  RequirementInfo="{'linktype_rmi_doors' '0000bab8 (/E-STEER Core/SubSystem Specifications/Application Functions/SF040A Motor Velocity)' '#SF040A_102' 'true' 'REQ:  SF040A_102' '' ; 'linktype_rmi_doors' '0000bab8 (/E-STEER Core/SubSystem Specifications/Application Functions/SF040A Motor Velocity)' '#SF040A_104' 'true' 'REQ:  SF040A_104' '' } %GIDa_70bdc363_1ace_4590_a213_a0f30a829861"
  Add1 : Sum  RequirementInfo="{'linktype_rmi_doors' '0000bab8 (/E-STEER Core/SubSystem Specifications/Application Functions/SF040A Motor Velocity)' '#SF040A_102' 'true' 'REQ:  SF040A_102' '' ; 'linktype_rmi_doors' '0000bab8 (/E-STEER Core/SubSystem Specifications/Application Functions/SF040A Motor Velocity)' '#SF040A_104' 'true' 'REQ:  SF040A_104' '' } %GIDa_c2db8d50_2946_46d9_85ab_cc3de1cc527e"  Inputs=+-
  Bitwise Operator1 : simulink/Logic and Bit Operations/Bitwise Operator  RequirementInfo="{'linktype_rmi_doors' '0000bab8 (/E-STEER Core/SubSystem Specifications/Application Functions/SF040A Motor Velocity)' '#SF040A_104' 'true' 'REQ:  SF040A_104' '' } %GIDa_70b53fa2_3671_4136_9201_409e5a9a2f29"  logicop=AND  UseBitMask=off  NumInputPorts=2  BitMask=bin2dec('')  BitMaskRealWorld=Stored Integer
  Bitwise Operator2 : simulink/Logic and Bit Operations/Bitwise Operator  RequirementInfo="{'linktype_rmi_doors' '0000bab8 (/E-STEER Core/SubSystem Specifications/Application Functions/SF040A Motor Velocity)' '#SF040A_102' 'true' 'REQ:  SF040A_102' '' ; 'linktype_rmi_doors' '0000bab8 (/E-STEER Core/SubSystem Specifications/Application Functions/SF040A Motor Velocity)' '#SF040A_104' 'true' 'REQ:  SF040A_104' '' } %GIDa_b156b9d0_05bd_47f3_a1d3_e6596e9f5baf"  logicop=AND  UseBitMask=off  NumInputPorts=2  BitMask=bin2dec('')  BitMaskRealWorld=Stored Integer
  Constant1 : Constant  Value=MOTVELMAXININVAL_CNT_U08
  CopyRight2 : Subsystem  Description=|  mask(Copyright Information){none=on}
      | Copyright info block.                                               
      |                                                                     
      | Place copyright information at the top of every subsystem in design.
      mask prompts: none "No parameters"
      mask help: Place copyright information at the top of every subsystem in design.
      mask Display:
      | NxtrConf = 'Nexteer Confidential';
      | 
      | sys = bdroot; %handle for the current model ("system")
      | first = get_param(sys,'Created');
      | first = first(end-3:end);  %year is last four digits
      | 
      | last = get_param(sys,'LastModifiedDate');
      | if isempty(last)
      |     last = datestr(now,'yyyy');
      | else
      |     last = last(end-3:end);
      | end
      | 
      | if strcmp(first,last)
      |     fprintf('%s -- Copyright %s Nexteer',NxtrConf,first)
      | else
      |     fprintf('%s -- %s%s- %s Nexteer',NxtrConf,char(169),first,last)
      | end
  Data Store Read : DataStoreRead  Priority=1  DataStoreName=MotAgBufPrev
  Data Store Read1 : DataStoreRead  Priority=1  DataStoreName=MotAgTiBufPrev
  Data Store Read2 : DataStoreRead  Priority=1  DataStoreName=MotAgBufIdxPrev
  Data Store Write : DataStoreWrite  Priority=2  DataStoreName=MotAgBufPrev
  Data Store Write1 : DataStoreWrite  Priority=2  DataStoreName=MotAgTiBufPrev
  Data Store Write2 : DataStoreWrite  Priority=2  DataStoreName=MotAgBufIdxPrev
  Data Type Conversion : DataTypeConversion  OutDataTypeStr=uint16
  Data Type Conversion1 : DataTypeConversion  OutDataTypeStr=single
  Data Type Conversion2 : DataTypeConversion  OutDataTypeStr=single
  If : If  RequirementInfo="{'linktype_rmi_doors' '0000bab8 (/E-STEER Core/SubSystem Specifications/Application Functions/SF040A Motor Velocity)' '#SF040A_111' 'true' 'REQ:  SF040A_111' '' } %GIDa_e06647f5_b1f4_4127_851c_c0596830fea9"  IfExpression=u1
  If1 : If  RequirementInfo="{'linktype_rmi_doors' '0000bab8 (/E-STEER Core/SubSystem Specifications/Application Functions/SF040A Motor Velocity)' '#SF040A_111' 'true' 'REQ:  SF040A_111' '' } %GIDa_6eac8974_23f8_47e7_a1a7_a4285d1b454a"  IfExpression=u1
  LimStat_f32 : NxtrLim/LimStat_f32  RequirementInfo="{'linktype_rmi_doors' '0000bab8 (/E-STEER Core/SubSystem Specifications/Application Functions/SF040A Motor Velocity)' '#SF040A_111' 'true' 'REQ:  SF040A_111' '' } %GIDa_646e0e96_5fe4_4319_8005_d07ee8e2d7b5"  LoLim=MOTVELMIN_MOTRADPERSEC_F32  HiLim=MOTVELMAX_MOTRADPERSEC_F32
      settings: AttributesFormatString=|
      | Low Limit: %<LoLim>
      | High Limit:%<HiLim>
  Merge : Merge  RequirementInfo="{'linktype_rmi_doors' '0000bab8 (/E-STEER Core/SubSystem Specifications/Application Functions/SF040A Motor Velocity)' '#SF040A_111' 'true' 'REQ:  SF040A_111' '' } %GIDa_e2bf39c5_c49a_417f_a966_2ae7208c09fc"
  Merge1 : Merge  RequirementInfo="{'linktype_rmi_doors' '0000bab8 (/E-STEER Core/SubSystem Specifications/Application Functions/SF040A Motor Velocity)' '#SF040A_111' 'true' 'REQ:  SF040A_111' '' } %GIDa_9e3b2446_b2fb_4c61_9f59_f25e82e8ef52"
  MotVelIninCntr : DataStoreRead  DataStoreName=MotVelIninCntr
  MotVelMotRefFrmDecision1 : Subsystem  RequirementInfo="{'linktype_rmi_doors' '0000bab8 (/E-STEER Core/SubSystem Specifications/Application Functions/SF040A Motor Velocity)' '#SF040A_111' 'true' 'REQ:  SF040A_111' '' } %GIDa_9ac65ac2_0a0c_4987_a5d2_b459b6618c75"  TreatAsAtomicUnit=on
  MotVelMotRefFrmDecision2 : Subsystem  RequirementInfo="{'linktype_rmi_doors' '0000bab8 (/E-STEER Core/SubSystem Specifications/Application Functions/SF040A Motor Velocity)' '#SF040A_111' 'true' 'REQ:  SF040A_111' '' } %GIDa_0599e73a_498e_4e23_9811_910be82f3cb3"  TreatAsAtomicUnit=on
  MotVelMrfDecision1 : Subsystem  RequirementInfo="{'linktype_rmi_doors' '0000bab8 (/E-STEER Core/SubSystem Specifications/Application Functions/SF040A Motor Velocity)' '#SF040A_111' 'true' 'REQ:  SF040A_111' '' } %GIDa_8f793b1d_da7d_4844_b94c_cbc372910247"  TreatAsAtomicUnit=on
  MotVelMrfDecision2 : Subsystem  RequirementInfo="{'linktype_rmi_doors' '0000bab8 (/E-STEER Core/SubSystem Specifications/Application Functions/SF040A Motor Velocity)' '#SF040A_111' 'true' 'REQ:  SF040A_111' '' } %GIDa_4aa3eebf_d918_4f49_a950_4d87e014101f"  TreatAsAtomicUnit=on
  Number of Delays : Constant  Value=BUFSIZE_CNT_U08  OutDataTypeStr=uint8
  Number of Delays1 : Constant  OutDataTypeStr=uint8
      settings: AttributesFormatString=%<OutDataTypeStr>
  Number of Delays10 : Constant  Value=ARCHGLBPRM_FLOATZEROTHD_ULS_F32
  Number of Delays11 : Constant  Value=BUFSIZECOMBD_CNT_U08  OutDataTypeStr=uint8
  Number of Delays2 : Constant  OutDataTypeStr=uint8
      settings: AttributesFormatString=%<OutDataTypeStr>
  Number of Delays4 : Constant  Value=BUFSIZECOMBD_CNT_U08  OutDataTypeStr=uint8
  Number of Delays5 : Constant  Value=0  OutDataTypeStr=uint32
      settings: AttributesFormatString=%<OutDataTypeStr>
  Number of Delays6 : Constant  Value=BUFSIZECOMBD_CNT_U08  OutDataTypeStr=uint8
  Number of Delays7 : Constant  Value=BITMASK16BIT_CNT_U32
  Number of Delays8 : Constant  Value=0  OutDataTypeStr=single
      settings: AttributesFormatString=%<OutDataTypeStr>
  Number of Delays9 : Constant  Value=0  OutDataTypeStr=single
      settings: AttributesFormatString=%<OutDataTypeStr>
  Product2 : Product  Inputs=*/  RndMeth=Zero
  Relational Operator : RelationalOperator  RequirementInfo="{'linktype_rmi_doors' '0000bab8 (/E-STEER Core/SubSystem Specifications/Application Functions/SF040A Motor Velocity)' '#SF040A_111' 'true' 'REQ:  SF040A_111' '' } %GIDa_ce3397b4_68d3_49e7_b3f8_01cee5f63783"  Operator=>  OutDataTypeStr=boolean
  Relational Operator1 : RelationalOperator  RequirementInfo="{'linktype_rmi_doors' '0000bab8 (/E-STEER Core/SubSystem Specifications/Application Functions/SF040A Motor Velocity)' '#SF040A_111' 'true' 'REQ:  SF040A_111' '' } %GIDa_33818d0b_4fe6_4be9_910b_3d2a8b00ec1e"  Operator=<  OutDataTypeStr=boolean
  Selector : Selector  RequirementInfo="{'linktype_rmi_doors' '0000bab8 (/E-STEER Core/SubSystem Specifications/Application Functions/SF040A Motor Velocity)' '#SF040A_102' 'true' 'REQ:  SF040A_102' '' } %GIDa_cdd3463f_e58b_40cc_9555_fe4bf37a239f"  IndexMode=Zero-based  InputPortWidth=16  IndexOptions=Index vector (port)  Indices=[1 3]  OutputSizes=1
  Selector1 : Selector  RequirementInfo="{'linktype_rmi_doors' '0000bab8 (/E-STEER Core/SubSystem Specifications/Application Functions/SF040A Motor Velocity)' '#SF040A_104' 'true' 'REQ:  SF040A_104' '' } %GIDa_a278e5a4_08da_42e7_af24_6c40370f2e21"  IndexMode=Zero-based  InputPortWidth=16  IndexOptions=Index vector (port)  Indices=[1 3]  OutputSizes=1
  SqdSumTiStampPrev : DataStoreMemory  DataStoreName=SqdSumTiStampPrev
  SqdSumTiStampPrev_Write : DataStoreWrite  DataStoreName=SqdSumTiStampPrev
  SumAg SqurdSum : Subsystem  TreatAsAtomicUnit=on
  SumAgTiMotRevSecPrev_Write : DataStoreWrite  DataStoreName=SumAgTiMotRevSecPrev
  SumAgTi_MotRevSecPrev : DataStoreMemory  DataStoreName=SumAgTiMotRevSecPrev
  SumTiStampBufSt : Subsystem  RequirementInfo="{'linktype_rmi_doors' '0000bab8 (/E-STEER Core/SubSystem Specifications/Application Functions/SF040A Motor Velocity)' '#SF040A_103' 'true' 'REQ:  SF040A_103' '' } %GIDa_3a3c0273_fd8a_41e4_b581_de4bde1370a4"  TreatAsAtomicUnit=on
  SumTiStampBufStPrev : DataStoreMemory  DataStoreName=SumTiStampBufStPrev  OutDataTypeStr=uint32
  SumTiStampBufStPrev_Write1 : DataStoreWrite  DataStoreName=SumTiStampBufStPrev
  Vector Concatenate : Concatenate
  Vector Concatenate1 : Concatenate
  dMotVelAvrgTi : DataStoreWrite  DataStoreName=dMotVelAvrgTi
  dMotVelMotAgRef : DataStoreWrite  DataStoreName=dMotVelMotAgRef
  dMotVelMotAgRef1 : DataStoreWrite  DataStoreName=dMotVelTiStampRef
  MotVelMrf : Outport
  wires:
  "MotAgBuf "/1 -> Vector Concatenate/2, Data Store Write/1
  Data Store Read/1 -> Vector Concatenate/1
  Vector Concatenate/1 -> [MotAgBuf], Selector/1
  MotAgTiBuf/1 -> Vector Concatenate1/2, Data Store Write1/1
  Data Store Read1/1 -> Vector Concatenate1/1
  Vector Concatenate1/1 -> SumTiStampBufSt/2(MotAgTiBuf), [MotAgTiBuf], Selector1/1
  Data Store Read2/1 -> Add/1
  Number of Delays2/1 -> Add/2
  Add/1 -> Bitwise Operator2/1
  Number of Delays/1 -> Add1/1
  Number of Delays1/1 -> Add1/2
  Add1/1 -> Bitwise Operator2/2
  Bitwise Operator2/1 -> Selector/2, Selector1/2
  Selector1/1 -> Bitwise Operator1/1
  Selector/1 -> dMotVelMotAgRef/1, [MotAgRef]
  Number of Delays7/1 -> Bitwise Operator1/2
  Bitwise Operator1/1 -> Data Type Conversion/1
  Data Type Conversion/1 -> SumAg SqurdSum/1(TiStampRef), Data Type Conversion2/1, SumTiStampBufSt/1(TiStampRef)
  Number of Delays11/1 -> SumTiStampBufSt/3(BufSizeCombd)
  Number of Delays5/1 -> SumTiStampBufStPrev_Write1/1
  Number of Delays4/1 -> Product2/2
  Product2/1 -> SumAg SqurdSum/6(AdjTiStampRef), Data Type Conversion1/1
  Number of Delays6/1 -> SumAg SqurdSum/2(BufSizeCombd)
  [MotAgRef] -> SumAg SqurdSum/5(MotAgRef)
  [MotAgBuf] -> SumAg SqurdSum/3(MotAgBuf)
  [MotAgTiBuf] -> SumAg SqurdSum/4(MotAgTiBuf)
  Number of Delays9/1 -> SumAgTiMotRevSecPrev_Write/1
  Number of Delays8/1 -> SqdSumTiStampPrev_Write/1
  SumAg SqurdSum/2(SumAgTi) -> [SumAgTi]
  SumAg SqurdSum/1(SqdSum) -> [SqdSum]
  [SqdSum] -> Relational Operator/1
  If/1 -> MotVelMrfDecision1/Action
  If/2 -> MotVelMrfDecision2/Action
  [SqdSum] -> MotVelMrfDecision1/2(SqdSum)
  [SumAgTi] -> MotVelMrfDecision1/1(SumAgTi)
  [SumAgTi] -> MotVelMrfDecision2/1(SumAgTi)
  MotVelMrfDecision2/1(MotVelMrf) -> Merge/2
  MotVelMrfDecision1/1(MotVelMrf) -> Merge/1
  Relational Operator/1 -> If/1
  Number of Delays10/1 -> Relational Operator/2
  MotVelIninCntr/1 -> Relational Operator1/1
  Constant1/1 -> Relational Operator1/2
  Merge/1 -> LimStat_f32/1
  If1/1 -> MotVelMotRefFrmDecision1/Action
  If1/2 -> MotVelMotRefFrmDecision2/Action
  LimStat_f32/1 -> MotVelMotRefFrmDecision2/1(MotVelMrf)
  MotVelMotRefFrmDecision2/1(MotVelMotRefFrm) -> Merge1/2
  MotVelMotRefFrmDecision1/1(MotVelMotRefFrm) -> Merge1/1
  Merge1/1 -> MotVelMrf/1
  SumTiStampBufSt/1(SumTiStampBufSt) -> Product2/1
  MotAgBufIdx/1 -> Data Store Write2/1
  Data Type Conversion2/1 -> dMotVelMotAgRef1/1
  Relational Operator1/1 -> If1/1
  Data Type Conversion1/1 -> dMotVelAvrgTi/1

== system SF040A_MotVel/MotVel/MotVelPer1/Indexing Counter/MotCtrlMotAgBufIdxReset/Copyright1 ==

== system SF040A_MotVel/MotVel/MotVelPer1/Indexing Counter/MotCtrlMotAgBufIdxSet/Copyright1 ==

== system SF040A_MotVel/MotVel/MotVelPer2/MtrVelMRFCalc/MtrVelMRFCalc/CopyRight2 ==

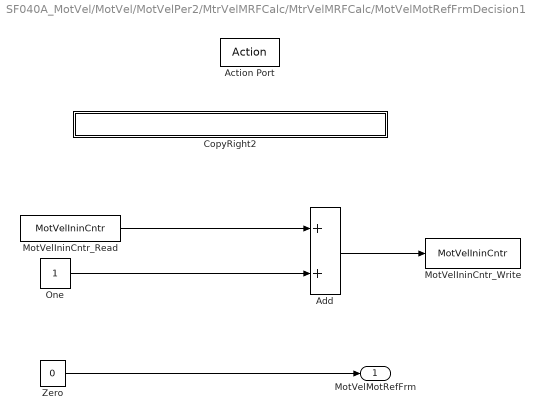
== system SF040A_MotVel/MotVel/MotVelPer2/MtrVelMRFCalc/MtrVelMRFCalc/MotVelMotRefFrmDecision1 ==
  Action Port : ActionPort  ActionType=then
  Add : Sum  OutDataTypeStr=Inherit: Inherit via back propagation
  CopyRight2 : Subsystem  Description=|  mask(Copyright Information){none=on}
      | Copyright info block.                                               
      |                                                                     
      | Place copyright information at the top of every subsystem in design.
      mask prompts: none "No parameters"
      mask help: Place copyright information at the top of every subsystem in design.
      mask Display:
      | NxtrConf = 'Nexteer Confidential';
      | 
      | sys = bdroot; %handle for the current model ("system")
      | first = get_param(sys,'Created');
      | first = first(end-3:end);  %year is last four digits
      | 
      | last = get_param(sys,'LastModifiedDate');
      | if isempty(last)
      |     last = datestr(now,'yyyy');
      | else
      |     last = last(end-3:end);
      | end
      | 
      | if strcmp(first,last)
      |     fprintf('%s -- Copyright %s Nexteer',NxtrConf,first)
      | else
      |     fprintf('%s -- %s%s- %s Nexteer',NxtrConf,char(169),first,last)
      | end
  MotVelIninCntr_Read : DataStoreRead  DataStoreName=MotVelIninCntr
  MotVelIninCntr_Write : DataStoreWrite  DataStoreName=MotVelIninCntr
  One : Constant  OutDataTypeStr=uint8
      settings: AttributesFormatString=%<OutDataTypeStr>
  Zero : Constant  Value=0  OutDataTypeStr=single
      settings: AttributesFormatString=%<OutDataTypeStr>
  MotVelMotRefFrm : Outport
  wires:
  Zero/1 -> MotVelMotRefFrm/1
  Add/1 -> MotVelIninCntr_Write/1
  One/1 -> Add/2
  MotVelIninCntr_Read/1 -> Add/1

== system SF040A_MotVel/MotVel/MotVelPer2/MtrVelMRFCalc/MtrVelMRFCalc/MotVelMotRefFrmDecision2 ==
  MotVelMrf : Inport
  Action Port : ActionPort  ActionType=else
  CopyRight2 : Subsystem  Description=|  mask(Copyright Information){none=on}
      | Copyright info block.                                               
      |                                                                     
      | Place copyright information at the top of every subsystem in design.
      mask prompts: none "No parameters"
      mask help: Place copyright information at the top of every subsystem in design.
      mask Display:
      | NxtrConf = 'Nexteer Confidential';
      | 
      | sys = bdroot; %handle for the current model ("system")
      | first = get_param(sys,'Created');
      | first = first(end-3:end);  %year is last four digits
      | 
      | last = get_param(sys,'LastModifiedDate');
      | if isempty(last)
      |     last = datestr(now,'yyyy');
      | else
      |     last = last(end-3:end);
      | end
      | 
      | if strcmp(first,last)
      |     fprintf('%s -- Copyright %s Nexteer',NxtrConf,first)
      | else
      |     fprintf('%s -- %s%s- %s Nexteer',NxtrConf,char(169),first,last)
      | end
  MotVelMotRefFrm : Outport
  wires:
  MotVelMrf/1 -> MotVelMotRefFrm/1
